simulink model "ghost_integrator"  (R2020b)
settings: Solver=FixedStepAuto  StartTime=0.0  StopTime=inf  FixedStep=0.02  RelTol=1e-3
undefined symbols (not defined in the file): DiscIntNeverNeededParam, Header, Point
libraries: robotlib x7
settings Model: Creator=safwan  LastModifiedBy=safwan
settings OptimizationCC: EnhancedBackFolding=on  PassReuseOutputArgsAs=Individual arguments  ZeroExternalMemoryAtStartup=off  ZeroInternalMemoryAtStartup=off  MaxStackSize=64  OptimizeBlockOrder=speed  DifferentSizesBufferReuse=on  OptimizationCustomize=off  EfficientTunableParamExpr=on
settings DebuggingCC: ParameterTunabilityLossMsg=error
settings HardwareCC: ProdBitPerPointer=32  ProdBitPerSizeT=32  ProdBitPerPtrDiffT=32  ProdLargestAtomicFloat=None  ProdIntDivRoundTo=Undefined  ProdEndianess=Unspecified  ProdWordSize=32  ProdHWDeviceType=Generic->Unspecified (assume 32-bit Generic)
settings SFSimCC: MATLABDynamicMemAlloc=off  SimTargetLang=C++
settings RTWCC: Description=Embedded Coder  SystemTargetFile=ert.tlc  HardwareBoard=Robot Operating System (ROS)  TLCOptions="-aInlineSetEventsForThisBaseRateFcn=TLC_FALSE -aSuppressMultiTaskScheduler=TLC_FALSE  -aRateBasedStepFcn=0"  TemplateMakefile=ert_default_tmf  Toolchain=Catkin  TargetLang=C++
settings CodeAppCC: ForceParamTrailComments=on  IgnoreCustomStorageClasses=off  OperatorAnnotations=on  SimulinkDataObjDesc=on  SFDataObjDesc=on  InsertBlockDesc=on

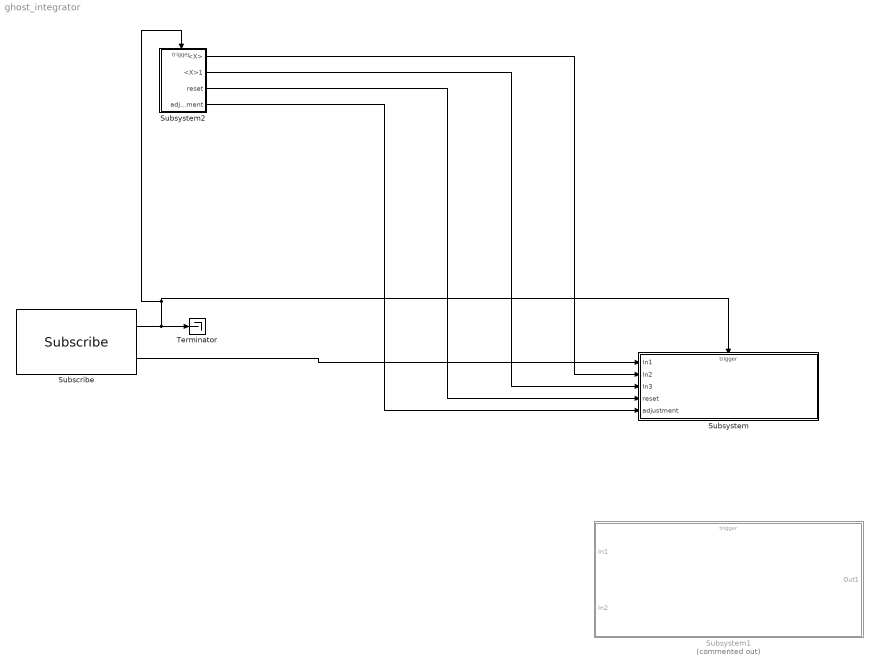
== system ghost_integrator ==
  Subscribe : robotlib/Subscribe  topicSource=Specify your own  topic=/ghost_vehicle/vel  messageType=geometry_msgs/TwistStamped  SampleTime=-1  legacyBusStruct=off  messageQueueLength=1
  Subsystem : Subsystem
  Subsystem1 : Subsystem  Commented=on
  Subsystem2 : Subsystem
  Terminator : Terminator
  wires:
  Subscribe/1 -> Subsystem2/Trigger, Subsystem/Trigger, Terminator/1
  Subscribe/2 -> Subsystem/1(In1)
  Subsystem2/1(<X>) -> Subsystem/2(In2)
  Subsystem2/2(<X>1) -> Subsystem/3(In3)
  Subsystem2/3(reset) -> Subsystem/4(reset)
  Subsystem2/4(adjustment) -> Subsystem/5(adjustment)

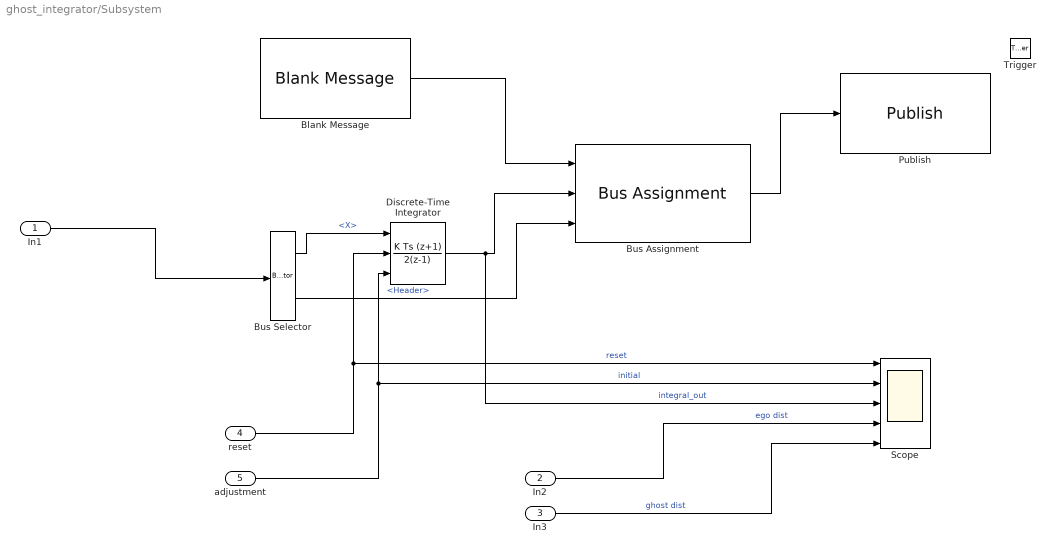
== system ghost_integrator/Subsystem ==
  In1 : Inport
  In2 : Inport  Port=2
  In3 : Inport  Port=3
  reset : Inport  Port=4
  adjustment : Inport  Port=5
  Trigger : TriggerPort  VariantControl=Variant  PortDimensions=1
  Blank Message : robotlib/Blank Message  messageClass=Message  entityType=geometry_msgs/PointStamped  messageType=geometry_msgs/PointStamped  SampleTime=-1  legacyBusStruct=off
  Bus Assignment : BusAssignment  AssignedSignals=Point.X,Header
  Bus Selector : BusSelector  OutputSignals=Twist.Linear.X,Header
  Discrete-Time Integrator : DiscreteIntegrator  IntegratorMethod=Integration: Trapezoidal  ExternalReset=rising  InitialConditionSource=external  SampleTime=-1  ICPrevOutput=DiscIntNeverNeededParam  ICPrevScaledInput=DiscIntNeverNeededParam
  Publish : robotlib/Publish  topicSource=Specify your own  topic=/ghost_dist_traveled  messageType=geometry_msgs/PointStamped  legacyBusStruct=off  messageQueueLength=1
  Scope : Scope  NumInputPorts=5
  wires:
  Bus Selector/2 -> Bus Assignment/3  "<Header>"
  In1/1 -> Bus Selector/1
  Bus Selector/1 -> Discrete-Time Integrator/1  "<X>"
  Bus Assignment/1 -> Publish/1
  Discrete-Time Integrator/1 -> Scope/3, Bus Assignment/2  "integral_out"
  Blank Message/1 -> Bus Assignment/1
  reset/1 -> Discrete-Time Integrator/2, Scope/1  "reset"
  adjustment/1 -> Discrete-Time Integrator/3, Scope/2  "initial"
  In2/1 -> Scope/4  "ego dist"
  In3/1 -> Scope/5  "ghost dist"

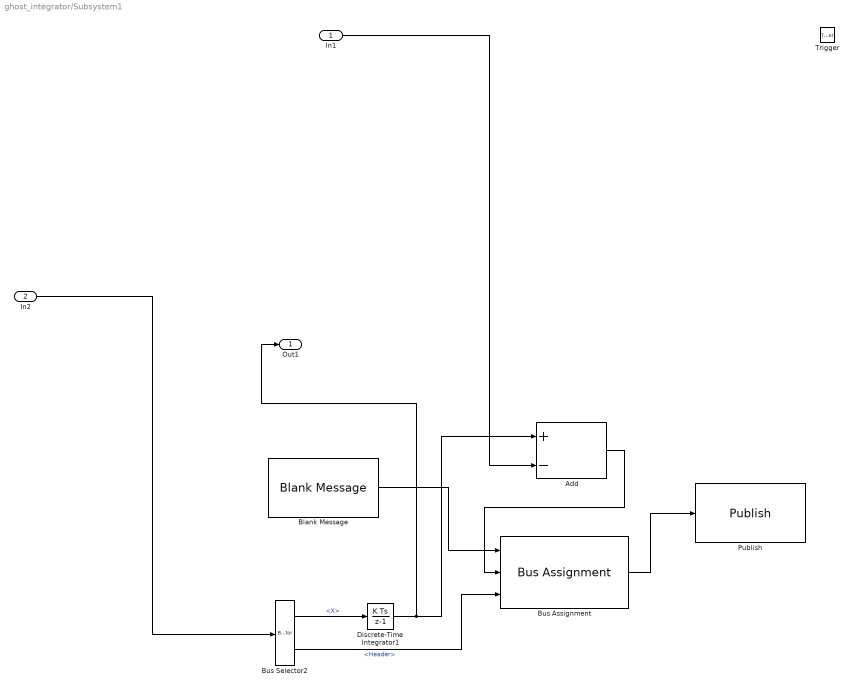
== system ghost_integrator/Subsystem1 ==
  In1 : Inport
  In2 : Inport  Port=2
  Trigger : TriggerPort  VariantControl=Variant  PortDimensions=1
  Add : Sum  Inputs=+-
  Blank Message : robotlib/Blank Message  messageClass=Message  entityType=geometry_msgs/PointStamped  messageType=geometry_msgs/PointStamped  SampleTime=-1  legacyBusStruct=off
  Bus Assignment : BusAssignment  AssignedSignals=Point.X,Header
  Bus Selector2 : BusSelector  OutputSignals=Twist.Linear.X,Header
  Discrete-Time Integrator1 : DiscreteIntegrator  SampleTime=-1  ICPrevOutput=DiscIntNeverNeededParam  ICPrevScaledInput=DiscIntNeverNeededParam
  Publish : robotlib/Publish  topicSource=Specify your own  topic=/ghost_dist_traveled  messageType=geometry_msgs/PointStamped  legacyBusStruct=off  messageQueueLength=1
  Out1 : Outport
  wires:
  Bus Selector2/2 -> Bus Assignment/3  "<Header>"
  In1/1 -> Add/2
  In2/1 -> Bus Selector2/1
  Add/1 -> Bus Assignment/2
  Blank Message/1 -> Bus Assignment/1
  Bus Selector2/1 -> Discrete-Time Integrator1/1  "<X>"
  Discrete-Time Integrator1/1 -> Out1/1, Add/1
  Bus Assignment/1 -> Publish/1

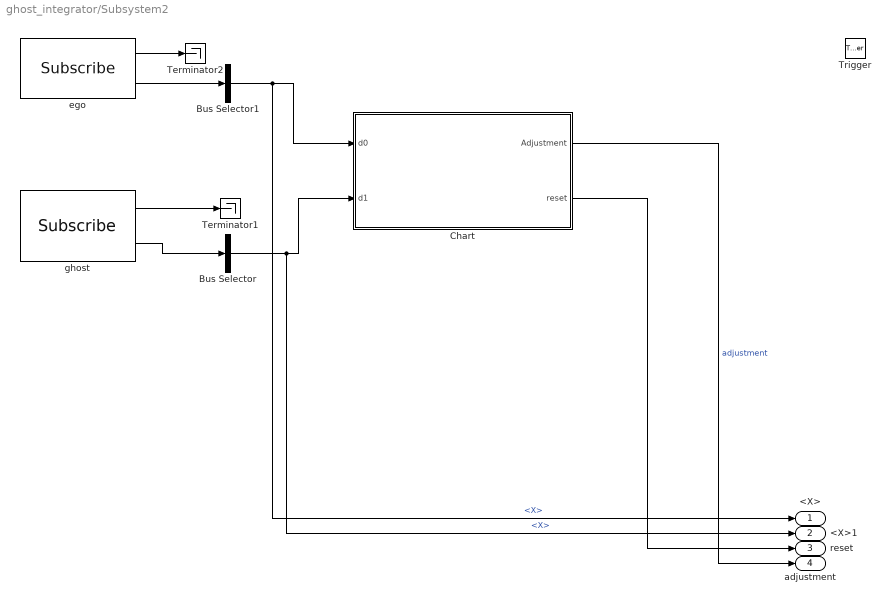
== system ghost_integrator/Subsystem2 ==
  Trigger : TriggerPort  VariantControl=Variant  PortDimensions=1
  Bus Selector : BusSelector  OutputSignals=Point.X
  Bus Selector1 : BusSelector  OutputSignals=Point.X
  Chart : Stateflow chart  TreatAsAtomicUnit=on
  Terminator1 : Terminator
  Terminator2 : Terminator
  ego : robotlib/Subscribe  topicSource=Specify your own  topic=/ego_dist_traveled  messageType=geometry_msgs/PointStamped  SampleTime=-1  legacyBusStruct=off  messageQueueLength=1
  ghost : robotlib/Subscribe  topicSource=Specify your own  topic=/ghost_dist_traveled  messageType=geometry_msgs/PointStamped  SampleTime=-1  legacyBusStruct=off  messageQueueLength=1
  <X> : Outport
  <X>1 : Outport  Port=2
  reset : Outport  Port=3
  adjustment : Outport  Port=4
  wires:
  ego/1 -> Terminator2/1
  Chart/1(Adjustment) -> adjustment/1  "adjustment"
  Chart/2(reset) -> reset/1
  ego/2 -> Bus Selector1/1
  Bus Selector/1 -> <X>1/1, Chart/2(d1)  "<X>"
  ghost/2 -> Bus Selector/1
  Bus Selector1/1 -> <X>/1, Chart/1(d0)  "<X>"
  ghost/1 -> Terminator1/1

== stateflow chart ghost_integrator/Subsystem2/Chart ==
  state State_2 [commented out]
    state sub1 [commented out]
    state sub2 [commented out]
      entry:reset=1;l=d0;
    (default) -> sub1 [commented out]
    sub1 -> sub2 [commented out] : [d1-d0 > 100.0]
  state idel [commented out]
    entry:reset=0;
  state startup
    entry:Adjustment=0;
  state catch_up
    entry: Adjustment=d0; reset=1;
    during:reset=1;
    exit: reset=0;
  state idle
  state slow_down
    entry: Adjustment=d0; reset=1;
    during:reset=1;
    exit: reset=0;
  (default) -> idel [commented out]
  idel -> State_2 [commented out] : after(30, sec)
  State_2 -> idel [commented out] : [d1-d0 < 100.0]
  catch_up -> idle
  (default) -> startup
  startup -> idle
  idle -> catch_up [order 1] : after(30,sec)[d1-d0 > 100]
  slow_down -> idle
  idle -> slow_down [order 2] : after(30,sec)[d1-d0 < 0]
  data: d0 input double; d1 input double; Adjustment output double size=1; reset output uint8
